simulink model "disc_linear_without_constant_member"  (R2023a)
settings: Solver=VariableStepAuto  StartTime=0.0  StopTime=70  RelTol=1e-3  EnableMultiTasking=on
model workspace (MAT data in the model file):
  Tp = 1
  u_liner = 1
settings Model: Creator=Laptop  LastModifiedBy=denys
settings SolverCC: AlgebraicLoopSolver=TrustRegion
settings DataIOCC: ReturnWorkspaceOutputs=off
settings OptimizationCC: LifeSpan=inf
settings DebuggingCC: UnconnectedInputMsg=warning  UnconnectedOutputMsg=warning  UnconnectedLineMsg=warning  SFUnexpectedBacktrackingDiag=warning  SFNoUnconditionalDefaultTransitionDiag=warning  ArithmeticOperatorsInVariantConditions=warning
settings ModelReferenceCC: EnableRefExpFcnMdlSchedulingChecks=on
settings SFSimCC: SimUseLocalCustomCode=off  CustomCodeUndefinedFunction=UseInterfaceOnly
settings RTWCC: RTWUseLocalCustomCode=off
settings CodeAppCC: StateflowObjectComments=on
settings GRTTargetCC: TargetLangStandard=C89/C90 (ANSI)
settings ConfigComp: CovMetricSettings=dw  CovSaveCumulativeToWorkspaceVar=on  CovSaveSingleToWorkspaceVar=on  CovExternalEMLEnable=off

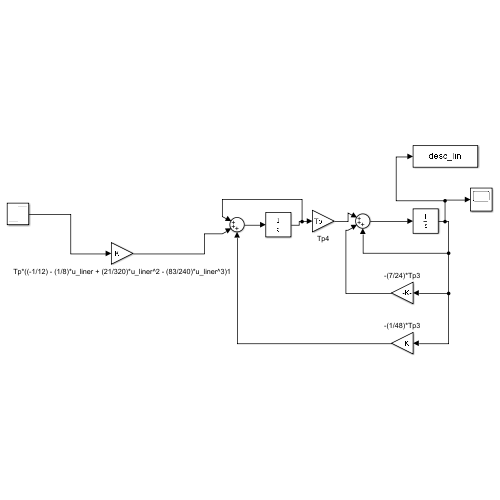
[thumbnail: Simulink's stored preview of the top-level diagram]
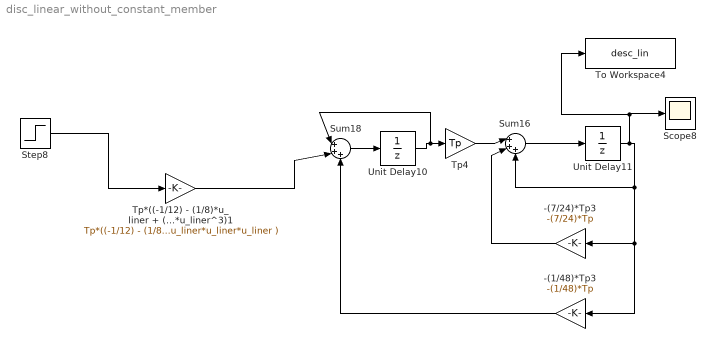
== system disc_linear_without_constant_member ==
  -(1/48)*Tp3 : Gain  Gain=-(1/48)*Tp
  -(7/24)*Tp3 : Gain  Gain=-(7/24)*Tp
  Scope8 : Scope
  Step8 : Step  SampleTime=Tp
  Sum16 : Sum  Inputs=|+++
  Sum18 : Sum  Inputs=|+++
  To Workspace4 : ToWorkspace  VariableName=desc_lin  SaveFormat=Timeseries  SampleTime=-1
  Tp*((-1/12) - (1/8)*u_liner + (21/320)*u_liner^2 - (83/240)*u_liner^3)1 : Gain  Gain=Tp*((-1/12) - (1/8)*u_liner + (21/320)*u_liner*u_liner - (83/240)*u_liner*u_liner*u_liner )
  Tp4 : Gain  Gain=Tp
  Unit Delay10 : UnitDelay  SampleTime=Tp  HasFrameUpgradeWarning=on
  Unit Delay11 : UnitDelay  SampleTime=Tp  HasFrameUpgradeWarning=on
  wires:
  Tp*((-1/12) - (1/8)*u_liner + (21/320)*u_liner^2 - (83/240)*u_liner^3)1/1 -> Sum18/2
  Sum18/1 -> Unit Delay10/1
  Unit Delay10/1 -> Sum18/1, Tp4/1
  Unit Delay11/1 -> To Workspace4/1, Scope8/1, -(1/48)*Tp3/1, -(7/24)*Tp3/1, Sum16/3
  Sum16/1 -> Unit Delay11/1
  Tp4/1 -> Sum16/1
  Step8/1 -> Tp*((-1/12) - (1/8)*u_liner + (21/320)*u_liner^2 - (83/240)*u_liner^3)1/1
  -(1/48)*Tp3/1 -> Sum18/3
  -(7/24)*Tp3/1 -> Sum16/2
